simulink model "test"  (R2020b)
settings: Solver=VariableStepAuto  StartTime=0.0  StopTime=1e3  RelTol=1e-3
libraries: component_lib x1
settings Model: Creator=Max  LastModifiedBy=Max

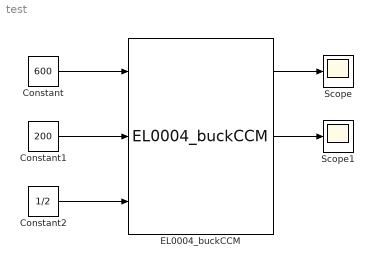
== system test ==
  Constant : Constant  Value=600
  Constant1 : Constant  Value=200
  Constant2 : Constant  Value=1/2
  EL0004_buckCCM : component_lib/Electrochemistry/EL0004_buckCCM  R=1e-3  C=10  L=1e-6  V_init=600
  Scope : Scope
  Scope1 : Scope
  wires:
  Constant/1 -> EL0004_buckCCM/1
  Constant1/1 -> EL0004_buckCCM/2
  Constant2/1 -> EL0004_buckCCM/3
  EL0004_buckCCM/1 -> Scope/1
  EL0004_buckCCM/2 -> Scope1/1
